simulink model "Reglare_PID_bun"  (R2023b)
settings: Solver=VariableStepAuto  StartTime=0.0  StopTime=10.0  RelTol=1e-3
values from neighbouring files (symbols this model uses):
  Kr_PID_chr1 = 0.6 * T_tangenta / (Tm1 * k)    (= 0.951998623616)    [Reglare_tangenta.m]
  Kr_PID_chr1_p = 0.95 * T_tangenta / (Tm1 * k)    (= 1.50733115406)    [Reglare_tangenta.m]
  Td_chr1 = 0.5 * Tm1    (= 4.935)    [Reglare_tangenta.m]
  Ti_PID_chr1 = Tm1    (= 9.87)    [Reglare_tangenta.m]
  Ti_PID_chr1_p = 2.4 * Tm1    (= 23.688)    [Reglare_tangenta.m]
undefined symbols (not defined in the file or in its folder): den_PID_chr0, den_PID_chr0_a, den_PID_chr1, den_PID_chr1_a, den_tangenta, num_PID_chr0, num_PID_chr0_a, num_PID_chr1, num_PID_chr1_a, num_tangenta
libraries: slpidlib x2
settings Model: Creator=raluc  LastModifiedBy=raluc

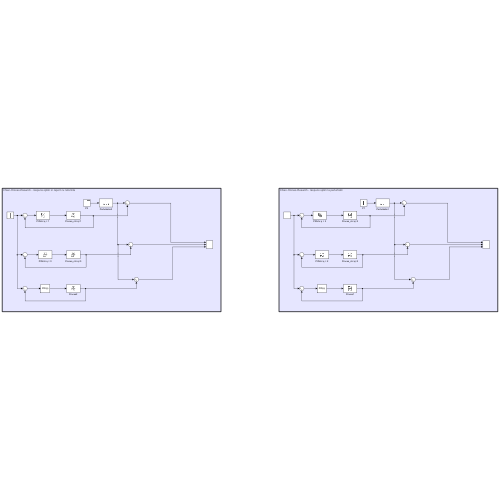
[thumbnail: Simulink's stored preview of the top-level diagram]
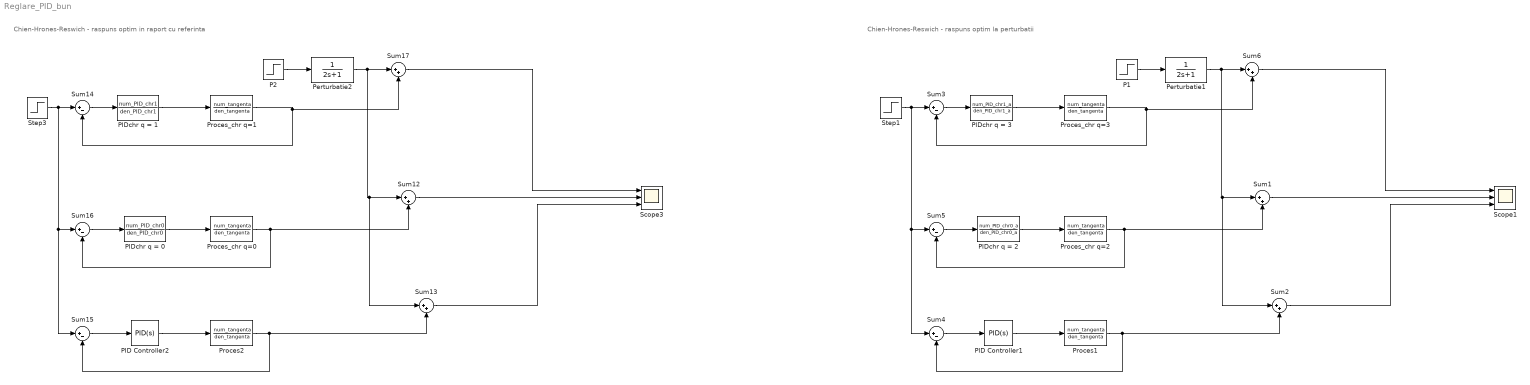
== system Reglare_PID_bun ==
  note: Chien-Hrones-Reswich - raspuns optim in raport cu referinta
  note: Chien-Hrones-Reswich - raspuns optim la perturbatii
  P1 : Step  SampleTime=0
  P2 : Step  SampleTime=0
  PID Controller1 : slpidlib/PID Controller  Controller=PID  Form=Parallel  TimeDomain=Continuous-time  UseExternalTs=off  SampleTime=-1  IntegratorMethod=Forward Euler  FilterMethod=Forward Euler  ControllerParametersSource=internal  P=Kr_PID_chr1_p  I=1/Ti_PID_chr1_p  UseKiTs=off  D=Td_chr1  N=100  UseFilter=on  TunerSelectOption=Transfer Function Based (PID Tuner App)  InitialConditionSource=internal  InitialConditionForIntegrator=0  InitialConditionForFilter=0  DifferentiatorICPrevScaledInput=0  ExternalReset=none  TrackingMode=off  Kt=1  LimitOutput=off  SatLimitsSource=internal  UpperSaturationLimit=inf  LowerSaturationLimit=-inf  LinearizeAsGain=on  AntiWindupMode=none  Kb=1  LimitIntegrator=off  UpperIntegratorSaturationLimit=inf  LowerIntegratorSaturationLimit=-inf  POutMin=[]  POutMax=[]  IOutMin=[]  IOutMax=[]  DOutMin=[]  DOutMax=[]  NOutMin=[]  NOutMax=[]  SumOutMin=[]  SumOutMax=[]  SaturationOutMin=[]  SaturationOutMax=[]  PParamMin=[]  PParamMax=[]  IParamMin=[]  IParamMax=[]  DParamMin=[]  DParamMax=[]  NParamMin=[]  NParamMax=[]  KbParamMin=[]  KbParamMax=[]  KtParamMin=[]  KtParamMax=[]  KbOutMin=[]  KbOutMax=[]  KtOutMin=[]  KtOutMax=[]  IntegratorOutMin=[]  IntegratorOutMax=[]  FilterOutMin=[]  FilterOutMax=[]  SumI1OutMin=[]  SumI1OutMax=[]  SumI2OutMin=[]  SumI2OutMax=[]  SumI3OutMin=[]  SumI3OutMax=[]  SumI4OutMin=[]  SumI4OutMax=[]  SumDOutMin=[]  SumDOutMax=[]  DifferentiatorOutMin=[]  DifferentiatorOutMax=[]  FilterDiffOutCoefMin=[]  FilterDiffOutCoefMax=[]  ReciprocalOutMin=[]  ReciprocalOutMax=[]  SumDenOutMin=[]  SumDenOutMax=[]  SumNumOutMin=[]  SumNumOutMax=[]  DivideOutMin=[]  DivideOutMax=[]  UdiffTsProdOutMin=[]  UdiffTsProdOutMax=[]  NTsProdOutMin=[]  NTsProdOutMax=[]  UintegralTsProdOutMin=[]  UintegralTsProdOutMax=[]  UngainTsProdOutMin=[]  UngainTsProdOutMax=[]  ClampingZeroOutDataTypeStr=Inherit: Inherit via back propagation  ClampingZeroOutMin=[]  ClampingZeroOutMax=[]  FilterDenConstantOutDataTypeStr=Inherit: Inherit via back propagation  FilterDenConstantOutMin=[]  FilterDenConstantOutMax=[]  PCopyOutDataTypeStr=Inherit: Inherit via back propagation  PCopyOutMin=[]  PCopyOutMax=[]  NCopyOutDataTypeStr=Inherit: Inherit via back propagation  NCopyOutMin=[]  NCopyOutMax=[]  IntegratorContinuousStateAttributes=''  IntegratorStateMustResolveToSignalObject=off  IntegratorRTWStateStorageClass=Auto  FilterContinuousStateAttributes=''  FilterStateMustResolveToSignalObject=off  FilterRTWStateStorageClass=Auto  ParallelPVariant=InternalParameters  IdealPVariant=Disabled  IVariant=InternalParameters  DVariant=InternalParameters  IntegratorVariant=Continuous  SatVariant=Disabled  AWVariant=Passthrough  PCopyVariant=Disabled  TRVariant=Disabled  FdbkBlocksVariant=Forward  IdealPFdbkVariant=Disabled  SatFdbkVariant=Disabled  DerivativeFilterVariant=ContFilter  NVariant=InternalParameters  NCopyVariant=Disabled  FilterICVariant=InternalICsFilter  IntegratorICVariant=InternalICs  ExternalResetVariant=Disabled  TRSumVariant=Passthrough  SumFdbkVariant=Disabled  SumVariant=Sum_PID  TsampFilterVariant=InternalTs  TsampNgainVariant=Passthrough  TsampIntegralVariant=Disabled_SignalSpec  ExternalSaturationOutDataTypeStr=Inherit: Same as second input
  PID Controller2 : slpidlib/PID Controller  Controller=PID  Form=Parallel  TimeDomain=Continuous-time  UseExternalTs=off  SampleTime=-1  IntegratorMethod=Forward Euler  FilterMethod=Forward Euler  ControllerParametersSource=internal  P=Kr_PID_chr1  I=1/Ti_PID_chr1  UseKiTs=off  D=Td_chr1  N=100  UseFilter=on  TunerSelectOption=Transfer Function Based (PID Tuner App)  InitialConditionSource=internal  InitialConditionForIntegrator=0  InitialConditionForFilter=0  DifferentiatorICPrevScaledInput=0  ExternalReset=none  TrackingMode=off  Kt=1  LimitOutput=off  SatLimitsSource=internal  UpperSaturationLimit=inf  LowerSaturationLimit=-inf  LinearizeAsGain=on  AntiWindupMode=none  Kb=1  LimitIntegrator=off  UpperIntegratorSaturationLimit=inf  LowerIntegratorSaturationLimit=-inf  POutMin=[]  POutMax=[]  IOutMin=[]  IOutMax=[]  DOutMin=[]  DOutMax=[]  NOutMin=[]  NOutMax=[]  SumOutMin=[]  SumOutMax=[]  SaturationOutMin=[]  SaturationOutMax=[]  PParamMin=[]  PParamMax=[]  IParamMin=[]  IParamMax=[]  DParamMin=[]  DParamMax=[]  NParamMin=[]  NParamMax=[]  KbParamMin=[]  KbParamMax=[]  KtParamMin=[]  KtParamMax=[]  KbOutMin=[]  KbOutMax=[]  KtOutMin=[]  KtOutMax=[]  IntegratorOutMin=[]  IntegratorOutMax=[]  FilterOutMin=[]  FilterOutMax=[]  SumI1OutMin=[]  SumI1OutMax=[]  SumI2OutMin=[]  SumI2OutMax=[]  SumI3OutMin=[]  SumI3OutMax=[]  SumI4OutMin=[]  SumI4OutMax=[]  SumDOutMin=[]  SumDOutMax=[]  DifferentiatorOutMin=[]  DifferentiatorOutMax=[]  FilterDiffOutCoefMin=[]  FilterDiffOutCoefMax=[]  ReciprocalOutMin=[]  ReciprocalOutMax=[]  SumDenOutMin=[]  SumDenOutMax=[]  SumNumOutMin=[]  SumNumOutMax=[]  DivideOutMin=[]  DivideOutMax=[]  UdiffTsProdOutMin=[]  UdiffTsProdOutMax=[]  NTsProdOutMin=[]  NTsProdOutMax=[]  UintegralTsProdOutMin=[]  UintegralTsProdOutMax=[]  UngainTsProdOutMin=[]  UngainTsProdOutMax=[]  ClampingZeroOutDataTypeStr=Inherit: Inherit via back propagation  ClampingZeroOutMin=[]  ClampingZeroOutMax=[]  FilterDenConstantOutDataTypeStr=Inherit: Inherit via back propagation  FilterDenConstantOutMin=[]  FilterDenConstantOutMax=[]  PCopyOutDataTypeStr=Inherit: Inherit via back propagation  PCopyOutMin=[]  PCopyOutMax=[]  NCopyOutDataTypeStr=Inherit: Inherit via back propagation  NCopyOutMin=[]  NCopyOutMax=[]  IntegratorContinuousStateAttributes=''  IntegratorStateMustResolveToSignalObject=off  IntegratorRTWStateStorageClass=Auto  FilterContinuousStateAttributes=''  FilterStateMustResolveToSignalObject=off  FilterRTWStateStorageClass=Auto  ParallelPVariant=InternalParameters  IdealPVariant=Disabled  IVariant=InternalParameters  DVariant=InternalParameters  IntegratorVariant=Continuous  SatVariant=Disabled  AWVariant=Passthrough  PCopyVariant=Disabled  TRVariant=Disabled  FdbkBlocksVariant=Forward  IdealPFdbkVariant=Disabled  SatFdbkVariant=Disabled  DerivativeFilterVariant=ContFilter  NVariant=InternalParameters  NCopyVariant=Disabled  FilterICVariant=InternalICsFilter  IntegratorICVariant=InternalICs  ExternalResetVariant=Disabled  TRSumVariant=Passthrough  SumFdbkVariant=Disabled  SumVariant=Sum_PID  TsampFilterVariant=InternalTs  TsampNgainVariant=Passthrough  TsampIntegralVariant=Disabled_SignalSpec  ExternalSaturationOutDataTypeStr=Inherit: Same as second input
  PIDchr q = 0 : TransferFcn  Numerator=num_PID_chr0  Denominator=den_PID_chr0
  PIDchr q = 1 : TransferFcn  Numerator=num_PID_chr1  Denominator=den_PID_chr1
  PIDchr q = 2 : TransferFcn  Numerator=num_PID_chr0_a  Denominator=den_PID_chr0_a
  PIDchr q = 3 : TransferFcn  Numerator=num_PID_chr1_a  Denominator=den_PID_chr1_a
  Perturbatie1 : TransferFcn  Denominator=[2 1]
  Perturbatie2 : TransferFcn  Denominator=[2 1]
  Proces1 : TransferFcn  Numerator=num_tangenta  Denominator=den_tangenta
  Proces2 : TransferFcn  Numerator=num_tangenta  Denominator=den_tangenta
  Proces_chr q={0..3} (4 alike) : TransferFcn  Numerator=num_tangenta  Denominator=den_tangenta
  Scope1 : Scope  NumInputPorts=3
  Scope3 : Scope  NumInputPorts=3
  Step1 : Step  After=10  SampleTime=0
  Step3 : Step  After=10  SampleTime=0
  Sum{1..2,6,12..13,17} (6 alike) : Sum  Inputs=|++
  Sum{3..5,14..16} (6 alike) : Sum  Inputs=|+-
  wires:
  PIDchr q = 0/1 -> Proces_chr q=0/1
  PID Controller2/1 -> Proces2/1
  Sum14/1 -> PIDchr q = 1/1
  Proces_chr q=0/1 -> Sum12/2, Sum16/2
  PIDchr q = 1/1 -> Proces_chr q=1/1
  Sum16/1 -> PIDchr q = 0/1
  Proces2/1 -> Sum13/2, Sum15/2
  Sum15/1 -> PID Controller2/1
  Step3/1 -> Sum15/1, Sum16/1, Sum14/1
  Perturbatie2/1 -> Sum13/1, Sum12/1, Sum17/1
  Proces_chr q=1/1 -> Sum17/2, Sum14/2
  P2/1 -> Perturbatie2/1
  Sum12/1 -> Scope3/2
  Sum13/1 -> Scope3/3
  Sum17/1 -> Scope3/1
  Sum2/1 -> Scope1/3
  Perturbatie1/1 -> Sum2/1, Sum1/1, Sum6/1
  P1/1 -> Perturbatie1/1
  Proces_chr q=3/1 -> Sum6/2, Sum3/2
  Sum1/1 -> Scope1/2
  Proces1/1 -> Sum2/2, Sum4/2
  Sum5/1 -> PIDchr q = 2/1
  Step1/1 -> Sum4/1, Sum5/1, Sum3/1
  Sum4/1 -> PID Controller1/1
  Sum3/1 -> PIDchr q = 3/1
  PIDchr q = 2/1 -> Proces_chr q=2/1
  PIDchr q = 3/1 -> Proces_chr q=3/1
  Sum6/1 -> Scope1/1
  Proces_chr q=2/1 -> Sum1/2, Sum5/2
  PID Controller1/1 -> Proces1/1
